simulink model "Research_project_CSTR_cascade"  (R2022b)
settings: Solver=ode23s  StartTime=0.0  StopTime=360  RelTol=1e-3
model workspace (MAT data in the model file):
  Var = 0
undefined symbols (not defined in the file): A, CA0, FA0, Tfeed, Tfeedout, Tj, U, V, v0, Xin, Xout
(part 1 of 2)
settings Model: Creator=ep740  LastModifiedBy=ep740

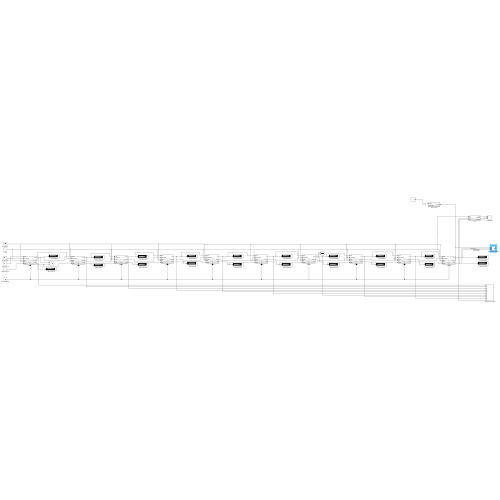
[thumbnail: Simulink's stored preview of the top-level diagram]
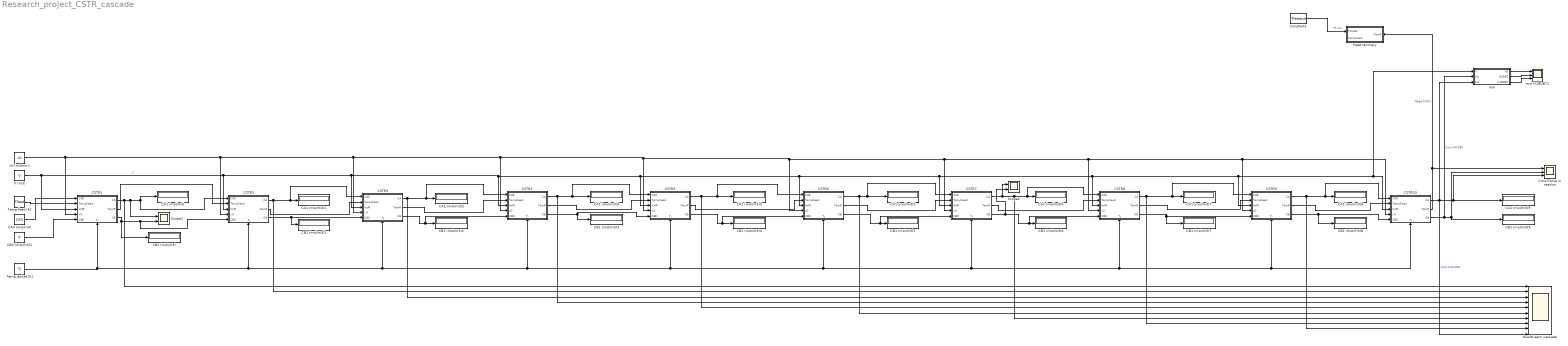
== system Research_project_CSTR_cascade ==
  CA0 (mol/m3) : Constant  Value=CA0
  CA1 (mol/m3){,1..9} (10 alike) : Display
  CB0 (mol/m3)1 : Constant  Value=0
  CB1 (mol/m3){,1..9} (10 alike) : Display
  CSTR1 : Subsystem
      settings: PortSchema="{\"entries\":[{\"content\":{\"sides\":[{\"content\":{\"connectorIds\":[\"In1\",\"In2\",\"In3\",\"In4\",\"In5\"]},\"type\":\"ConnectorPlacement.EquallySpacedRectSide\",\"uuid\":\"eea4af67-33e6-4bfc-a396-c7a4a079851b\"},{\"content\":{\"connectorIds\":[\"Out1\",\"Out2\",\"Out3\"],\"side\":\"RIGHT\"},\"type\":\"ConnectorPlacement.EquallySpacedRectSide\",\"uuid\":\"f422c120-f512-47db-9acf-190dfdbb71b1\"},{\"content\":{\"connectorIds\":[],\"side\":\"TOP\"},\"type\":\"ConnectorPlacement.EquallySpacedRectSide\",\"uuid\":\"a25ad9e8-8239-4679-905d-cedaf00f41ce\"},{\"content\":{\"connectorIds\":[\"In6\"],\"side\":\"BOTTOM\"},\"type\":\"ConnectorPlacement.EquallySpacedRectSide\",\"uuid\":\"a59362ac-e6e7-47b6-87e1-dd90c06e84db\"}]},\"type\":\"ConnectorPlacement.EquallySpacedConnector\",\"uuid\":\"827fa9d5-9d21-4e75-ac02-d0df13947b6d\"}],\"packageUris\":[\"http://schema.mathworks.com/mf0/Connector/R2020b\"],\"version\":\"1.0\"}"
  CSTR10 : Subsystem
      settings: PortSchema="{\"entries\":[{\"content\":{\"sides\":[{\"content\":{\"connectorIds\":[\"In1\",\"In2\",\"In3\",\"In4\",\"In5\"]},\"type\":\"ConnectorPlacement.EquallySpacedRectSide\",\"uuid\":\"eea4af67-33e6-4bfc-a396-c7a4a079851b\"},{\"content\":{\"connectorIds\":[\"Out1\",\"Out2\",\"Out3\"],\"side\":\"RIGHT\"},\"type\":\"ConnectorPlacement.EquallySpacedRectSide\",\"uuid\":\"f422c120-f512-47db-9acf-190dfdbb71b1\"},{\"content\":{\"connectorIds\":[],\"side\":\"TOP\"},\"type\":\"ConnectorPlacement.EquallySpacedRectSide\",\"uuid\":\"a25ad9e8-8239-4679-905d-cedaf00f41ce\"},{\"content\":{\"connectorIds\":[\"In6\"],\"side\":\"BOTTOM\"},\"type\":\"ConnectorPlacement.EquallySpacedRectSide\",\"uuid\":\"a59362ac-e6e7-47b6-87e1-dd90c06e84db\"}]},\"type\":\"ConnectorPlacement.EquallySpacedConnector\",\"uuid\":\"827fa9d5-9d21-4e75-ac02-d0df13947b6d\"}],\"packageUris\":[\"http://schema.mathworks.com/mf0/Connector/R2020b\"],\"version\":\"1.0\"}"
  CSTR2 : Subsystem
      settings: PortSchema="{\"entries\":[{\"content\":{\"sides\":[{\"content\":{\"connectorIds\":[\"In1\",\"In2\",\"In3\",\"In4\",\"In5\"]},\"type\":\"ConnectorPlacement.EquallySpacedRectSide\",\"uuid\":\"eea4af67-33e6-4bfc-a396-c7a4a079851b\"},{\"content\":{\"connectorIds\":[\"Out1\",\"Out2\",\"Out3\"],\"side\":\"RIGHT\"},\"type\":\"ConnectorPlacement.EquallySpacedRectSide\",\"uuid\":\"f422c120-f512-47db-9acf-190dfdbb71b1\"},{\"content\":{\"connectorIds\":[],\"side\":\"TOP\"},\"type\":\"ConnectorPlacement.EquallySpacedRectSide\",\"uuid\":\"a25ad9e8-8239-4679-905d-cedaf00f41ce\"},{\"content\":{\"connectorIds\":[\"In6\"],\"side\":\"BOTTOM\"},\"type\":\"ConnectorPlacement.EquallySpacedRectSide\",\"uuid\":\"a59362ac-e6e7-47b6-87e1-dd90c06e84db\"}]},\"type\":\"ConnectorPlacement.EquallySpacedConnector\",\"uuid\":\"827fa9d5-9d21-4e75-ac02-d0df13947b6d\"}],\"packageUris\":[\"http://schema.mathworks.com/mf0/Connector/R2020b\"],\"version\":\"1.0\"}"
  CSTR3 : Subsystem
      settings: PortSchema="{\"entries\":[{\"content\":{\"sides\":[{\"content\":{\"connectorIds\":[\"In1\",\"In2\",\"In3\",\"In4\",\"In5\"]},\"type\":\"ConnectorPlacement.EquallySpacedRectSide\",\"uuid\":\"eea4af67-33e6-4bfc-a396-c7a4a079851b\"},{\"content\":{\"connectorIds\":[\"Out1\",\"Out2\",\"Out3\"],\"side\":\"RIGHT\"},\"type\":\"ConnectorPlacement.EquallySpacedRectSide\",\"uuid\":\"f422c120-f512-47db-9acf-190dfdbb71b1\"},{\"content\":{\"connectorIds\":[],\"side\":\"TOP\"},\"type\":\"ConnectorPlacement.EquallySpacedRectSide\",\"uuid\":\"a25ad9e8-8239-4679-905d-cedaf00f41ce\"},{\"content\":{\"connectorIds\":[\"In6\"],\"side\":\"BOTTOM\"},\"type\":\"ConnectorPlacement.EquallySpacedRectSide\",\"uuid\":\"a59362ac-e6e7-47b6-87e1-dd90c06e84db\"}]},\"type\":\"ConnectorPlacement.EquallySpacedConnector\",\"uuid\":\"827fa9d5-9d21-4e75-ac02-d0df13947b6d\"}],\"packageUris\":[\"http://schema.mathworks.com/mf0/Connector/R2020b\"],\"version\":\"1.0\"}"
  CSTR4 : Subsystem
      settings: PortSchema="{\"entries\":[{\"content\":{\"sides\":[{\"content\":{\"connectorIds\":[\"In1\",\"In2\",\"In3\",\"In4\",\"In5\"]},\"type\":\"ConnectorPlacement.EquallySpacedRectSide\",\"uuid\":\"eea4af67-33e6-4bfc-a396-c7a4a079851b\"},{\"content\":{\"connectorIds\":[\"Out1\",\"Out2\",\"Out3\"],\"side\":\"RIGHT\"},\"type\":\"ConnectorPlacement.EquallySpacedRectSide\",\"uuid\":\"f422c120-f512-47db-9acf-190dfdbb71b1\"},{\"content\":{\"connectorIds\":[],\"side\":\"TOP\"},\"type\":\"ConnectorPlacement.EquallySpacedRectSide\",\"uuid\":\"a25ad9e8-8239-4679-905d-cedaf00f41ce\"},{\"content\":{\"connectorIds\":[\"In6\"],\"side\":\"BOTTOM\"},\"type\":\"ConnectorPlacement.EquallySpacedRectSide\",\"uuid\":\"a59362ac-e6e7-47b6-87e1-dd90c06e84db\"}]},\"type\":\"ConnectorPlacement.EquallySpacedConnector\",\"uuid\":\"827fa9d5-9d21-4e75-ac02-d0df13947b6d\"}],\"packageUris\":[\"http://schema.mathworks.com/mf0/Connector/R2020b\"],\"version\":\"1.0\"}"
  CSTR5 : Subsystem
      settings: PortSchema="{\"entries\":[{\"content\":{\"sides\":[{\"content\":{\"connectorIds\":[\"In1\",\"In2\",\"In3\",\"In4\",\"In5\"]},\"type\":\"ConnectorPlacement.EquallySpacedRectSide\",\"uuid\":\"eea4af67-33e6-4bfc-a396-c7a4a079851b\"},{\"content\":{\"connectorIds\":[\"Out1\",\"Out2\",\"Out3\"],\"side\":\"RIGHT\"},\"type\":\"ConnectorPlacement.EquallySpacedRectSide\",\"uuid\":\"f422c120-f512-47db-9acf-190dfdbb71b1\"},{\"content\":{\"connectorIds\":[],\"side\":\"TOP\"},\"type\":\"ConnectorPlacement.EquallySpacedRectSide\",\"uuid\":\"a25ad9e8-8239-4679-905d-cedaf00f41ce\"},{\"content\":{\"connectorIds\":[\"In6\"],\"side\":\"BOTTOM\"},\"type\":\"ConnectorPlacement.EquallySpacedRectSide\",\"uuid\":\"a59362ac-e6e7-47b6-87e1-dd90c06e84db\"}]},\"type\":\"ConnectorPlacement.EquallySpacedConnector\",\"uuid\":\"827fa9d5-9d21-4e75-ac02-d0df13947b6d\"}],\"packageUris\":[\"http://schema.mathworks.com/mf0/Connector/R2020b\"],\"version\":\"1.0\"}"
  CSTR6 : Subsystem
      settings: PortSchema="{\"entries\":[{\"content\":{\"sides\":[{\"content\":{\"connectorIds\":[\"In1\",\"In2\",\"In3\",\"In4\",\"In5\"]},\"type\":\"ConnectorPlacement.EquallySpacedRectSide\",\"uuid\":\"eea4af67-33e6-4bfc-a396-c7a4a079851b\"},{\"content\":{\"connectorIds\":[\"Out1\",\"Out2\",\"Out3\"],\"side\":\"RIGHT\"},\"type\":\"ConnectorPlacement.EquallySpacedRectSide\",\"uuid\":\"f422c120-f512-47db-9acf-190dfdbb71b1\"},{\"content\":{\"connectorIds\":[],\"side\":\"TOP\"},\"type\":\"ConnectorPlacement.EquallySpacedRectSide\",\"uuid\":\"a25ad9e8-8239-4679-905d-cedaf00f41ce\"},{\"content\":{\"connectorIds\":[\"In6\"],\"side\":\"BOTTOM\"},\"type\":\"ConnectorPlacement.EquallySpacedRectSide\",\"uuid\":\"a59362ac-e6e7-47b6-87e1-dd90c06e84db\"}]},\"type\":\"ConnectorPlacement.EquallySpacedConnector\",\"uuid\":\"827fa9d5-9d21-4e75-ac02-d0df13947b6d\"}],\"packageUris\":[\"http://schema.mathworks.com/mf0/Connector/R2020b\"],\"version\":\"1.0\"}"
  CSTR7 : Subsystem
      settings: PortSchema="{\"entries\":[{\"content\":{\"sides\":[{\"content\":{\"connectorIds\":[\"In1\",\"In2\",\"In3\",\"In4\",\"In5\"]},\"type\":\"ConnectorPlacement.EquallySpacedRectSide\",\"uuid\":\"eea4af67-33e6-4bfc-a396-c7a4a079851b\"},{\"content\":{\"connectorIds\":[\"Out1\",\"Out2\",\"Out3\"],\"side\":\"RIGHT\"},\"type\":\"ConnectorPlacement.EquallySpacedRectSide\",\"uuid\":\"f422c120-f512-47db-9acf-190dfdbb71b1\"},{\"content\":{\"connectorIds\":[],\"side\":\"TOP\"},\"type\":\"ConnectorPlacement.EquallySpacedRectSide\",\"uuid\":\"a25ad9e8-8239-4679-905d-cedaf00f41ce\"},{\"content\":{\"connectorIds\":[\"In6\"],\"side\":\"BOTTOM\"},\"type\":\"ConnectorPlacement.EquallySpacedRectSide\",\"uuid\":\"a59362ac-e6e7-47b6-87e1-dd90c06e84db\"}]},\"type\":\"ConnectorPlacement.EquallySpacedConnector\",\"uuid\":\"827fa9d5-9d21-4e75-ac02-d0df13947b6d\"}],\"packageUris\":[\"http://schema.mathworks.com/mf0/Connector/R2020b\"],\"version\":\"1.0\"}"
  CSTR8 : Subsystem
      settings: PortSchema="{\"entries\":[{\"content\":{\"sides\":[{\"content\":{\"connectorIds\":[\"In1\",\"In2\",\"In3\",\"In4\",\"In5\"]},\"type\":\"ConnectorPlacement.EquallySpacedRectSide\",\"uuid\":\"eea4af67-33e6-4bfc-a396-c7a4a079851b\"},{\"content\":{\"connectorIds\":[\"Out1\",\"Out2\",\"Out3\"],\"side\":\"RIGHT\"},\"type\":\"ConnectorPlacement.EquallySpacedRectSide\",\"uuid\":\"f422c120-f512-47db-9acf-190dfdbb71b1\"},{\"content\":{\"connectorIds\":[],\"side\":\"TOP\"},\"type\":\"ConnectorPlacement.EquallySpacedRectSide\",\"uuid\":\"a25ad9e8-8239-4679-905d-cedaf00f41ce\"},{\"content\":{\"connectorIds\":[\"In6\"],\"side\":\"BOTTOM\"},\"type\":\"ConnectorPlacement.EquallySpacedRectSide\",\"uuid\":\"a59362ac-e6e7-47b6-87e1-dd90c06e84db\"}]},\"type\":\"ConnectorPlacement.EquallySpacedConnector\",\"uuid\":\"827fa9d5-9d21-4e75-ac02-d0df13947b6d\"}],\"packageUris\":[\"http://schema.mathworks.com/mf0/Connector/R2020b\"],\"version\":\"1.0\"}"
  CSTR9 : Subsystem
      settings: PortSchema="{\"entries\":[{\"content\":{\"sides\":[{\"content\":{\"connectorIds\":[\"In1\",\"In2\",\"In3\",\"In4\",\"In5\"]},\"type\":\"ConnectorPlacement.EquallySpacedRectSide\",\"uuid\":\"eea4af67-33e6-4bfc-a396-c7a4a079851b\"},{\"content\":{\"connectorIds\":[\"Out1\",\"Out2\",\"Out3\"],\"side\":\"RIGHT\"},\"type\":\"ConnectorPlacement.EquallySpacedRectSide\",\"uuid\":\"f422c120-f512-47db-9acf-190dfdbb71b1\"},{\"content\":{\"connectorIds\":[],\"side\":\"TOP\"},\"type\":\"ConnectorPlacement.EquallySpacedRectSide\",\"uuid\":\"a25ad9e8-8239-4679-905d-cedaf00f41ce\"},{\"content\":{\"connectorIds\":[\"In6\"],\"side\":\"BOTTOM\"},\"type\":\"ConnectorPlacement.EquallySpacedRectSide\",\"uuid\":\"a59362ac-e6e7-47b6-87e1-dd90c06e84db\"}]},\"type\":\"ConnectorPlacement.EquallySpacedConnector\",\"uuid\":\"827fa9d5-9d21-4e75-ac02-d0df13947b6d\"}],\"packageUris\":[\"http://schema.mathworks.com/mf0/Connector/R2020b\"],\"version\":\"1.0\"}"
  Conc/Temp in reactor : Scope  NumInputPorts=3
  Constant1 : Constant  Value=Tfeedout
  Heat recovery : Subsystem
      settings: PortSchema="{\"entries\":[{\"content\":{\"sides\":[{\"content\":{\"connectorIds\":[\"In1\",\"Out1\"]},\"type\":\"ConnectorPlacement.EquallySpacedRectSide\",\"uuid\":\"573787ca-756b-47b8-a520-c4bb68d941bf\"},{\"content\":{\"connectorIds\":[\"In2\"],\"side\":\"RIGHT\"},\"type\":\"ConnectorPlacement.EquallySpacedRectSide\",\"uuid\":\"b1db1cb3-615d-4df7-8934-c0c48918d084\"},{\"content\":{\"connectorIds\":[],\"side\":\"TOP\"},\"type\":\"ConnectorPlacement.EquallySpacedRectSide\",\"uuid\":\"ffba5464-70c2-446d-94e9-0aafb3934113\"},{\"content\":{\"connectorIds\":[],\"side\":\"BOTTOM\"},\"type\":\"ConnectorPlacement.EquallySpacedRectSide\",\"uuid\":\"d4927b64-3679-4f6a-88f6-0667a528553b\"}]},\"type\":\"ConnectorPlacement.EquallySpacedConnector\",\"uuid\":\"96bf0ad9-972e-429c-80b4-1b1cb34767e8\"}],\"packageUris\":[\"http://schema.mathworks.com/mf0/Connector/R2020b\"],\"version\":\"1.0\"}"
  Scope1 : Scope  NumInputPorts=2
  Scope2 : Scope  NumInputPorts=2
  Temp Jacket (K) : Constant  Value=Tj
  Temp feed (K) : Constant  Value=Tfeed
  V (m3) : Constant  Value=V
  dCa/dt each cascade : Scope  NumInputPorts=10
  mol : Subsystem
  mol H18DBT1 : Scope  NumInputPorts=3
  v0 (m3/min) : Constant  Value=v0  VectorParams1D=off
  wires:
  CA0 (mol/m3)/1 -> CSTR1/1(CA0)
  CB0 (mol/m3)1/1 -> CSTR1/5(CB0)
  CSTR1/1(CA) -> dCa/dt each cascade/1, CSTR2/1(CA0), CA1 (mol/m3)/1, Scope1/1
  CSTR1/3(CB) -> CB1 (mol/m3)/1, CSTR2/5(CB0), Scope1/2
  V (m3)/1 -> CSTR2/3(VolR), CSTR3/3(VolR), CSTR4/3(VolR), CSTR5/3(VolR), CSTR6/3(VolR), CSTR7/3(VolR), CSTR8/3(VolR), CSTR9/3(VolR), CSTR10/3(VolR), mol/1(V), CSTR1/3(VolR)  "V"
  v0 (m3/min)/1 -> CSTR1/4(v0), CSTR2/4(v0), CSTR3/4(v0), CSTR4/4(v0), CSTR5/4(v0), CSTR6/4(v0), CSTR7/4(v0), CSTR8/4(v0), CSTR10/4(v0), CSTR9/4(v0)
  CSTR2/1(CA) -> dCa/dt each cascade/2, CSTR3/1(CA0), CA1 (mol/m3)1/1
  CSTR2/3(CB) -> CSTR3/5(CB0), CB1 (mol/m3)1/1
  CSTR1/2(TemR) -> CSTR2/2(TempFeed)
  CSTR3/3(CB) -> CSTR4/5(CB0), CB1 (mol/m3)2/1
  CSTR3/1(CA) -> dCa/dt each cascade/3, CSTR4/1(CA0), CA1 (mol/m3)2/1
  CSTR2/2(TemR) -> CSTR3/2(TempFeed)
  CSTR3/2(TemR) -> CSTR4/2(TempFeed)
  CSTR4/1(CA) -> dCa/dt each cascade/4, CSTR5/1(CA0), CA1 (mol/m3)3/1
  CSTR4/3(CB) -> CSTR5/5(CB0), CB1 (mol/m3)3/1
  CSTR5/3(CB) -> CSTR6/5(CB0), CB1 (mol/m3)4/1
  CSTR5/1(CA) -> dCa/dt each cascade/5, CSTR6/1(CA0), CA1 (mol/m3)4/1
  CSTR4/2(TemR) -> CSTR5/2(TempFeed)
  CSTR6/3(CB) -> CSTR7/5(CB0), CB1 (mol/m3)5/1
  CSTR6/1(CA) -> dCa/dt each cascade/6, CSTR7/1(CA0), CA1 (mol/m3)5/1
  CSTR5/2(TemR) -> CSTR6/2(TempFeed)
  CSTR6/2(TemR) -> CSTR7/2(TempFeed)
  CSTR7/1(CA) -> Scope2/1, dCa/dt each cascade/7, CSTR8/1(CA0), CA1 (mol/m3)6/1
  CSTR7/3(CB) -> Scope2/2, CSTR8/5(CB0), CB1 (mol/m3)6/1
  CSTR8/1(CA) -> dCa/dt each cascade/8, CSTR9/1(CA0), CA1 (mol/m3)7/1
  CSTR8/3(CB) -> CSTR9/5(CB0), CB1 (mol/m3)7/1
  CSTR7/2(TemR) -> CSTR8/2(TempFeed)
  CSTR9/3(CB) -> CSTR10/5(CB0), CB1 (mol/m3)8/1
  CSTR9/1(CA) -> dCa/dt each cascade/9, CSTR10/1(CA0), CA1 (mol/m3)8/1
  CSTR8/2(TemR) -> CSTR9/2(TempFeed)
  CSTR10/3(CB) -> mol/2(Cb), Conc/Temp in reactor/2, CB1 (mol/m3)9/1  "Conc H0-DBT"
  CSTR10/1(CA) -> mol/3(CA), dCa/dt each cascade/10, Conc/Temp in reactor/3, CA1 (mol/m3)9/1  "Conc H18-DBT"
  CSTR9/2(TemR) -> CSTR10/2(TempFeed)
  Temp Jacket (K)/1 -> CSTR2/6(Tj), CSTR3/6(Tj), CSTR4/6(Tj), CSTR5/6(Tj), CSTR6/6(Tj), CSTR7/6(Tj), CSTR8/6(Tj), CSTR10/6(Tj), CSTR9/6(Tj), CSTR1/6(Tj)
  CSTR10/2(TemR) -> Heat recovery/2(TemR), Conc/Temp in reactor/1  "Tfeed 573K)"
  Constant1/1 -> Heat recovery/1(Toutlet)  "Tf out"
  Temp feed (K)/1 -> CSTR1/2(TempFeed)
  mol/1(H2) -> mol H18DBT1/1
  mol/2(H0DBT) -> mol H18DBT1/2
  mol/3(H18DBT) -> mol H18DBT1/3

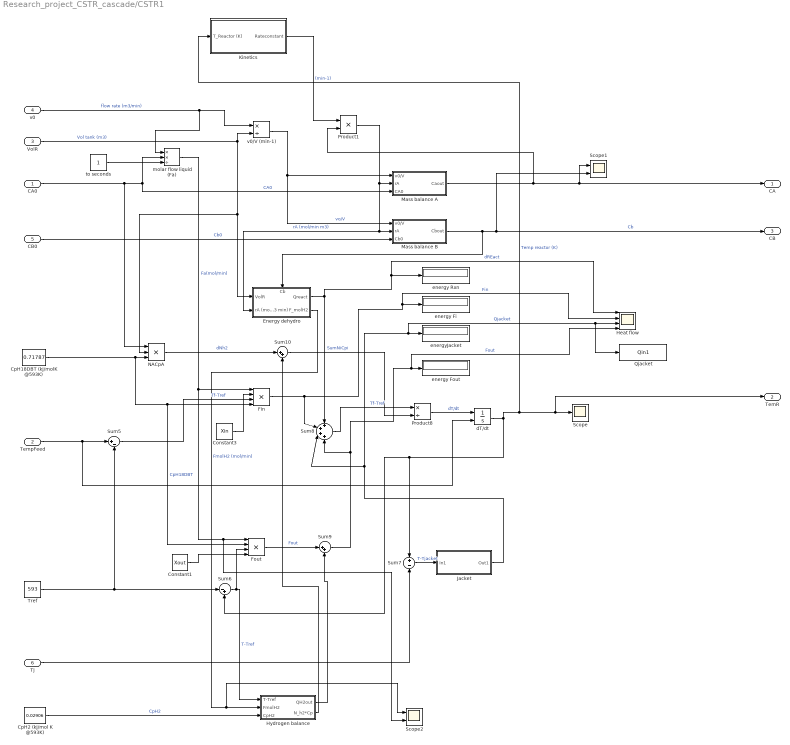
== system Research_project_CSTR_cascade/CSTR1 ==
  CA0 : Inport
  TempFeed : Inport  Port=2
  VolR : Inport  Port=3
  v0 : Inport  Port=4
  CB0 : Inport  Port=5
  Tj : Inport  Port=6
  Constant1 : Constant  Value=Xout
  Constant3 : Constant  Value=Xin
  CpH18DBT (kj/molK @593K) : Constant  Value=0.71787
  CpH2 (kj/mol K @593K) : Constant  Value=0.02906
  Energy dehydro : Subsystem
      settings: PortSchema="{\"entries\":[{\"content\":{\"sides\":[{\"content\":{\"connectorIds\":[\"In1\",\"In2\"]},\"type\":\"ConnectorPlacement.EquallySpacedRectSide\",\"uuid\":\"ea2ca829-97b9-403b-8ba1-0454ae3e30fe\"},{\"content\":{\"connectorIds\":[\"Out1\",\"Out2\"],\"side\":\"RIGHT\"},\"type\":\"ConnectorPlacement.EquallySpacedRectSide\",\"uuid\":\"58c9b242-3f0e-4d7f-8153-41ceacc042f7\"},{\"content\":{\"connectorIds\":[\"In3\"],\"side\":\"TOP\"},\"type\":\"ConnectorPlacement.EquallySpacedRectSide\",\"uuid\":\"130a98c9-d360-4861-8a60-9ab6de0c7020\"}]},\"type\":\"ConnectorPlacement.EquallySpacedConnector\",\"uuid\":\"a36fbf0c-f6b7-4cf9-83b8-7faebe270894\"}],\"packageUris\":[\"http://schema.mathworks.com/mf0/Connector/R2020b\"],\"version\":\"1.0\"}"
  Fin : Product  Inputs=4
  Fout : Product  Inputs=4
  Heat flow : Scope  NumInputPorts=4
  Hydrogen balance : Subsystem
  Jacket : Subsystem
  Kinetics : Subsystem
  Mass balance A : Subsystem
  Mass balance B : Subsystem
  NACpA : Product  Inputs=3
  Product1 : Product
  Product8 : Product  Inputs=*/
  Qjacket : ToWorkspace  VariableName=Qin1  SaveFormat=Timeseries  SampleTime=1
  Scope : Scope
  Scope1 : Scope  NumInputPorts=2
  Scope2 : Scope  NumInputPorts=2
  Sum10 : Sum  Inputs=|++
  Sum5 : Sum  Inputs=|+-
  Sum6 : Sum  Inputs=|-+
  Sum7 : Sum  Inputs=+-
  Sum8 : Sum  Inputs=++++
  Sum9 : Sum  Inputs=|++
  Tref : Constant  Value=593
  dT/dt : Integrator  InitialConditionSource=external  InitialCondition=593
  energy Fi : Display
  energy Fout : Display
  energy Rxn : Display
  energyJacket : Display
  molar flow liquid (Fa) : Product  Inputs=**/
  to seconds : Constant
  v0/V (min-1) : Product  Inputs=*/
  CA : Outport
  TemR : Outport  Port=2
  CB : Outport  Port=3
  wires:
  VolR/1 -> Energy dehydro/1(VolR), NACpA/2, v0/V (min-1)/2  "Vol tank (m3)"
  v0/1 -> v0/V (min-1)/1, molar flow liquid (Fa)/1  "flow rate (m3/min)"
  CA0/1 -> NACpA/1, molar flow liquid (Fa)/2, Mass balance A/3(CA0)  "CA0"
  Product1/1 -> Mass balance A/2(rA), Energy dehydro/2(rA (mol/m3 min)), Mass balance B/2(rA)  "rA (mol/min m3)"
  CB0/1 -> Mass balance B/3(Cb0)  "Cb0"
  v0/V (min-1)/1 -> Mass balance B/1(v0/V), Mass balance A/1(v0/V)  "vo/V"
  Mass balance B/1(Cbout) -> CB/1, Scope1/2, Energy dehydro/3(Cb)  "Cb"
  CpH18DBT (kj/molK @593K)/1 -> NACpA/3, Fin/4, Fout/2  "CpH18DBT"
  Tref/1 -> Sum5/2, Sum6/1
  Sum5/1 -> Fin/3  "Tf-Tref"
  to seconds/1 -> molar flow liquid (Fa)/3
  molar flow liquid (Fa)/1 -> Scope2/2, Fout/1, Fin/1  "Fa(mol/min)"
  dT/dt/1 -> Kinetics/1(T_Reactor (K)), TemR/1, Scope/1, Sum6/2, Sum7/1  "Temp reactor (K)"
  Sum6/1 -> Hydrogen balance/1(T-Tref), Fout/3  "T-Tref"
  Tj/1 -> Sum7/2
  Jacket/1(Out1) -> Qjacket/1, Heat flow/3, energyJacket/1, Sum8/3  "Qjacket"
  Fin/1 -> Heat flow/2, energy Fi/1, Sum8/2  "Fin"
  Sum9/1 -> Heat flow/4, energy Fout/1, Sum8/4  "Fout"
  Energy dehydro/1(Qreact) -> Sum8/1, Heat flow/1, energy Rxn/1  "dREact"
  Sum8/1 -> Product8/1  "Tf-Tref"
  Product8/1 -> dT/dt/1  "dT/dt"
  Constant1/1 -> Fout/4
  TempFeed/1 -> dT/dt/2, Sum5/1
  Kinetics/1(Rateconstant) -> Product1/1  "(min-1)"
  Constant3/1 -> Fin/2
  CpH2 (kj/mol K @593K)/1 -> Hydrogen balance/3(CpH2)  "CpH2"
  Energy dehydro/2(F_molH2) -> Scope2/1, Hydrogen balance/2(FmolH2)  "FmolH2 (mol/min)"
  Fout/1 -> Sum9/1  "Fout"
  Sum7/1 -> Jacket/1(In1)  "T-Tjacket"
  Hydrogen balance/1(QH2out) -> Sum9/2
  NACpA/1 -> Sum10/1  "dNh2"
  Sum10/1 -> Product8/2  "SumNiCpi"
  Hydrogen balance/2(N_h2*Cp) -> Sum10/2
  Mass balance A/1(Caout) -> Scope1/1, CA/1, Product1/2

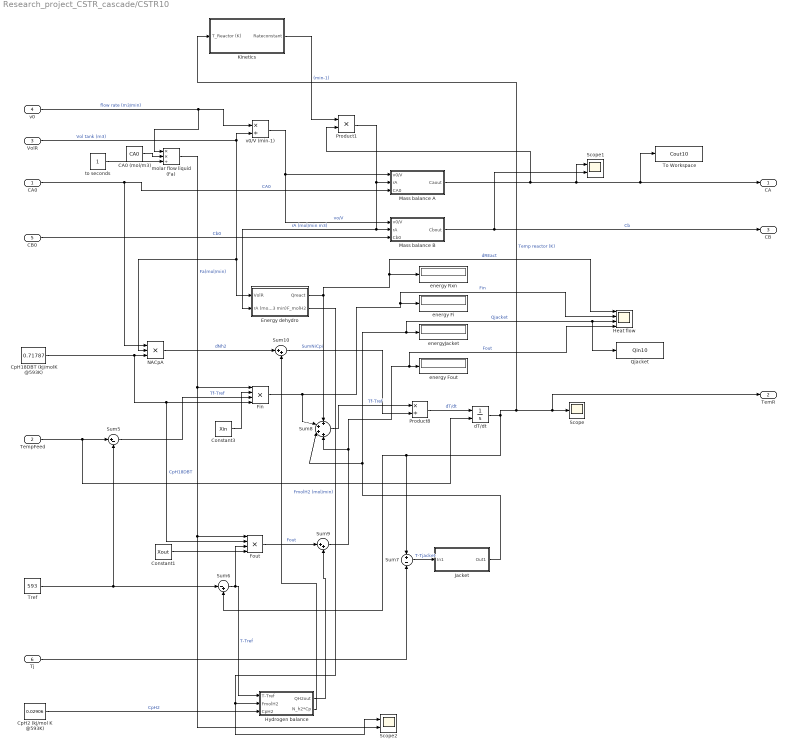
== system Research_project_CSTR_cascade/CSTR10 ==
  CA0 : Inport
  TempFeed : Inport  Port=2
  VolR : Inport  Port=3
  v0 : Inport  Port=4
  CB0 : Inport  Port=5
  Tj : Inport  Port=6
  CA0 (mol/m3) : Constant  Value=CA0
  Constant1 : Constant  Value=Xout
  Constant3 : Constant  Value=Xin
  CpH18DBT (kj/molK @593K) : Constant  Value=0.71787
  CpH2 (kj/mol K @593K) : Constant  Value=0.02906
  Energy dehydro : Subsystem
  Fin : Product  Inputs=4
  Fout : Product  Inputs=4
  Heat flow : Scope  NumInputPorts=4
  Hydrogen balance : Subsystem
  Jacket : Subsystem
  Kinetics : Subsystem
  Mass balance A : Subsystem
  Mass balance B : Subsystem
  NACpA : Product  Inputs=3
  Product1 : Product
  Product8 : Product  Inputs=*/
  Qjacket : ToWorkspace  VariableName=Qin10  SaveFormat=Timeseries  SampleTime=1
  Scope : Scope
  Scope1 : Scope  NumInputPorts=2
  Scope2 : Scope  NumInputPorts=2
  Sum10 : Sum  Inputs=|++
  Sum5 : Sum  Inputs=|+-
  Sum6 : Sum  Inputs=|-+
  Sum7 : Sum  Inputs=+-
  Sum8 : Sum  Inputs=++++
  Sum9 : Sum  Inputs=|++
  To Workspace : ToWorkspace  VariableName=Cout10  SaveFormat=Timeseries  SampleTime=5
  Tref : Constant  Value=593
  dT/dt : Integrator  InitialConditionSource=external  InitialCondition=593
  energy Fi : Display
  energy Fout : Display
  energy Rxn : Display
  energyJacket : Display
  molar flow liquid (Fa) : Product  Inputs=**/
  to seconds : Constant
  v0/V (min-1) : Product  Inputs=*/
  CA : Outport
  TemR : Outport  Port=2
  CB : Outport  Port=3
  wires:
  VolR/1 -> Energy dehydro/1(VolR), NACpA/2, v0/V (min-1)/2  "Vol tank (m3)"
  v0/1 -> v0/V (min-1)/1, molar flow liquid (Fa)/1  "flow rate (m3/min)"
  CA0/1 -> NACpA/1, Mass balance A/3(CA0)  "CA0"
  Product1/1 -> Mass balance A/2(rA), Energy dehydro/2(rA (mol/m3 min)), Mass balance B/2(rA)  "rA (mol/min m3)"
  CB0/1 -> Mass balance B/3(Cb0)  "Cb0"
  v0/V (min-1)/1 -> Mass balance B/1(v0/V), Mass balance A/1(v0/V)  "vo/V"
  Mass balance B/1(Cbout) -> CB/1, Scope1/2  "Cb"
  CpH18DBT (kj/molK @593K)/1 -> NACpA/3, Fin/4, Fout/2  "CpH18DBT"
  Tref/1 -> Sum5/2, Sum6/1
  Sum5/1 -> Fin/3  "Tf-Tref"
  to seconds/1 -> molar flow liquid (Fa)/3
  dT/dt/1 -> Kinetics/1(T_Reactor (K)), TemR/1, Scope/1, Sum6/2, Sum7/1  "Temp reactor (K)"
  Sum6/1 -> Hydrogen balance/1(T-Tref), Fout/3  "T-Tref"
  Tj/1 -> Sum7/2
  Jacket/1(Out1) -> Qjacket/1, Heat flow/3, energyJacket/1, Sum8/3  "Qjacket"
  Fin/1 -> Heat flow/2, energy Fi/1, Sum8/2  "Fin"
  Sum9/1 -> Heat flow/4, energy Fout/1, Sum8/4  "Fout"
  Energy dehydro/1(Qreact) -> Sum8/1, Heat flow/1, energy Rxn/1  "dREact"
  Sum8/1 -> Product8/1  "Tf-Tref"
  Product8/1 -> dT/dt/1  "dT/dt"
  Constant1/1 -> Fout/4
  TempFeed/1 -> dT/dt/2, Sum5/1
  Kinetics/1(Rateconstant) -> Product1/1  "(min-1)"
  Constant3/1 -> Fin/2
  CpH2 (kj/mol K @593K)/1 -> Hydrogen balance/3(CpH2)  "CpH2"
  Energy dehydro/2(F_molH2) -> Scope2/1, Hydrogen balance/2(FmolH2)  "FmolH2 (mol/min)"
  Fout/1 -> Sum9/1  "Fout"
  Sum7/1 -> Jacket/1(In1)  "T-Tjacket"
  Hydrogen balance/1(QH2out) -> Sum9/2
  NACpA/1 -> Sum10/1  "dNh2"
  Sum10/1 -> Product8/2  "SumNiCpi"
  Hydrogen balance/2(N_h2*Cp) -> Sum10/2
  Mass balance A/1(Caout) -> Scope1/1, To Workspace/1, CA/1, Product1/2
  CA0 (mol/m3)/1 -> molar flow liquid (Fa)/2
  molar flow liquid (Fa)/1 -> Fin/1, Fout/1, Scope2/2  "Fa(mol/min)"

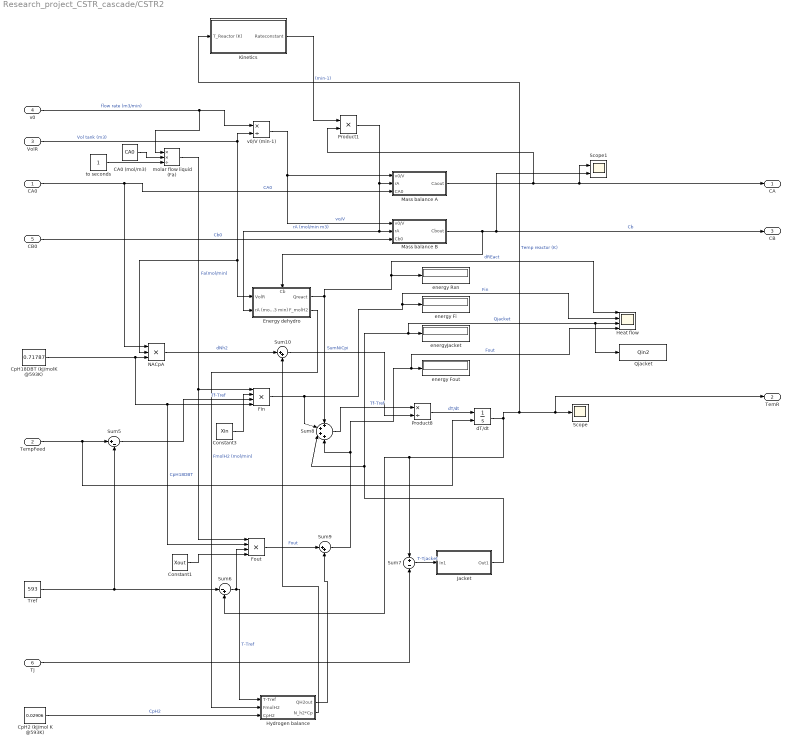
== system Research_project_CSTR_cascade/CSTR2 ==
  CA0 : Inport
  TempFeed : Inport  Port=2
  VolR : Inport  Port=3
  v0 : Inport  Port=4
  CB0 : Inport  Port=5
  Tj : Inport  Port=6
  CA0 (mol/m3) : Constant  Value=CA0
  Constant1 : Constant  Value=Xout
  Constant3 : Constant  Value=Xin
  CpH18DBT (kj/molK @593K) : Constant  Value=0.71787
  CpH2 (kj/mol K @593K) : Constant  Value=0.02906
  Energy dehydro : Subsystem
      settings: PortSchema="{\"entries\":[{\"content\":{\"sides\":[{\"content\":{\"connectorIds\":[\"In1\",\"In2\"]},\"type\":\"ConnectorPlacement.EquallySpacedRectSide\",\"uuid\":\"ea2ca829-97b9-403b-8ba1-0454ae3e30fe\"},{\"content\":{\"connectorIds\":[\"Out1\",\"Out2\"],\"side\":\"RIGHT\"},\"type\":\"ConnectorPlacement.EquallySpacedRectSide\",\"uuid\":\"58c9b242-3f0e-4d7f-8153-41ceacc042f7\"},{\"content\":{\"connectorIds\":[\"In3\"],\"side\":\"TOP\"},\"type\":\"ConnectorPlacement.EquallySpacedRectSide\",\"uuid\":\"130a98c9-d360-4861-8a60-9ab6de0c7020\"}]},\"type\":\"ConnectorPlacement.EquallySpacedConnector\",\"uuid\":\"a36fbf0c-f6b7-4cf9-83b8-7faebe270894\"}],\"packageUris\":[\"http://schema.mathworks.com/mf0/Connector/R2020b\"],\"version\":\"1.0\"}"
  Fin : Product  Inputs=4
  Fout : Product  Inputs=4
  Heat flow : Scope  NumInputPorts=4
  Hydrogen balance : Subsystem
  Jacket : Subsystem
  Kinetics : Subsystem
  Mass balance A : Subsystem
  Mass balance B : Subsystem
  NACpA : Product  Inputs=3
  Product1 : Product
  Product8 : Product  Inputs=*/
  Qjacket : ToWorkspace  VariableName=Qin2  SaveFormat=Timeseries  SampleTime=1
  Scope : Scope
  Scope1 : Scope  NumInputPorts=2
  Sum10 : Sum  Inputs=|++
  Sum5 : Sum  Inputs=|+-
  Sum6 : Sum  Inputs=|-+
  Sum7 : Sum  Inputs=+-
  Sum8 : Sum  Inputs=++++
  Sum9 : Sum  Inputs=|++
  Tref : Constant  Value=593
  dT/dt : Integrator  InitialConditionSource=external  InitialCondition=593
  energy Fi : Display
  energy Fout : Display
  energy Rxn : Display
  energyJacket : Display
  molar flow liquid (Fa) : Product  Inputs=**/
  to seconds : Constant
  v0/V (min-1) : Product  Inputs=*/
  CA : Outport
  TemR : Outport  Port=2
  CB : Outport  Port=3
  wires:
  VolR/1 -> Energy dehydro/1(VolR), NACpA/2, v0/V (min-1)/2  "Vol tank (m3)"
  v0/1 -> v0/V (min-1)/1, molar flow liquid (Fa)/1  "flow rate (m3/min)"
  CA0/1 -> NACpA/1, Mass balance A/3(CA0)  "CA0"
  Product1/1 -> Mass balance A/2(rA), Energy dehydro/2(rA (mol/m3 min)), Mass balance B/2(rA)  "rA (mol/min m3)"
  CB0/1 -> Mass balance B/3(Cb0)  "Cb0"
  v0/V (min-1)/1 -> Mass balance B/1(v0/V), Mass balance A/1(v0/V)  "vo/V"
  Mass balance B/1(Cbout) -> CB/1, Scope1/2, Energy dehydro/3(Cb)  "Cb"
  CpH18DBT (kj/molK @593K)/1 -> NACpA/3, Fin/4, Fout/2  "CpH18DBT"
  Tref/1 -> Sum5/2, Sum6/1
  Sum5/1 -> Fin/3  "Tf-Tref"
  to seconds/1 -> molar flow liquid (Fa)/3
  molar flow liquid (Fa)/1 -> Fout/1, Fin/1  "Fa(mol/min)"
  dT/dt/1 -> Kinetics/1(T_Reactor (K)), TemR/1, Scope/1, Sum6/2, Sum7/1  "Temp reactor (K)"
  Sum6/1 -> Hydrogen balance/1(T-Tref), Fout/3  "T-Tref"
  Tj/1 -> Sum7/2
  Jacket/1(Out1) -> Qjacket/1, Heat flow/3, energyJacket/1, Sum8/3  "Qjacket"
  Fin/1 -> Heat flow/2, energy Fi/1, Sum8/2  "Fin"
  Sum9/1 -> Heat flow/4, energy Fout/1, Sum8/4  "Fout"
  Energy dehydro/1(Qreact) -> Sum8/1, Heat flow/1, energy Rxn/1  "dREact"
  Sum8/1 -> Product8/1  "Tf-Tref"
  Product8/1 -> dT/dt/1  "dT/dt"
  Constant1/1 -> Fout/4
  TempFeed/1 -> dT/dt/2, Sum5/1
  Kinetics/1(Rateconstant) -> Product1/1  "(min-1)"
  Constant3/1 -> Fin/2
  CpH2 (kj/mol K @593K)/1 -> Hydrogen balance/3(CpH2)  "CpH2"
  Energy dehydro/2(F_molH2) -> Hydrogen balance/2(FmolH2)  "FmolH2 (mol/min)"
  Fout/1 -> Sum9/1  "Fout"
  Sum7/1 -> Jacket/1(In1)  "T-Tjacket"
  Hydrogen balance/1(QH2out) -> Sum9/2
  NACpA/1 -> Sum10/1  "dNh2"
  Sum10/1 -> Product8/2  "SumNiCpi"
  Hydrogen balance/2(N_h2*Cp) -> Sum10/2
  Mass balance A/1(Caout) -> Scope1/1, CA/1, Product1/2
  CA0 (mol/m3)/1 -> molar flow liquid (Fa)/2

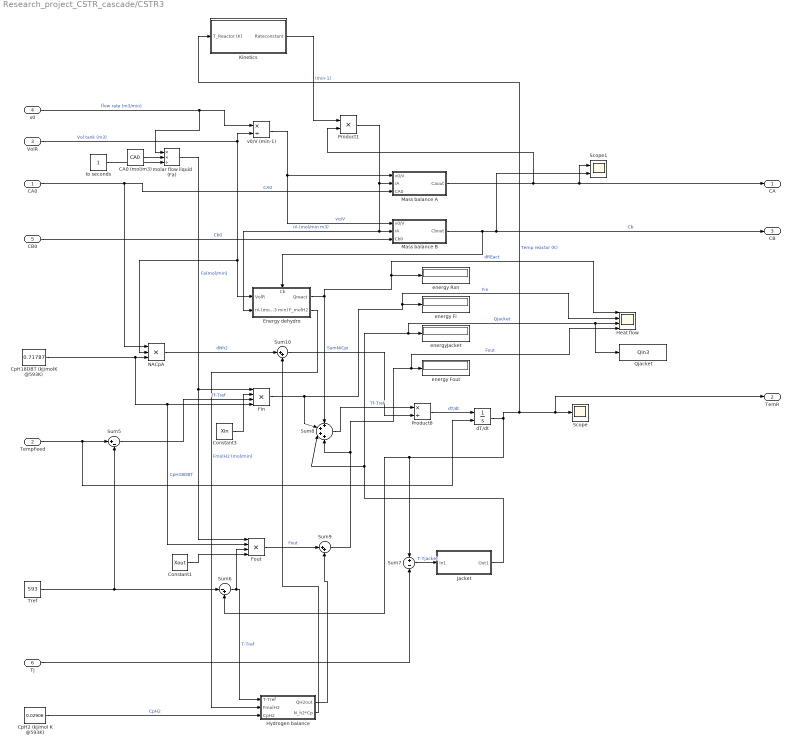
== system Research_project_CSTR_cascade/CSTR3 ==
  CA0 : Inport
  TempFeed : Inport  Port=2
  VolR : Inport  Port=3
  v0 : Inport  Port=4
  CB0 : Inport  Port=5
  Tj : Inport  Port=6
  CA0 (mol/m3) : Constant  Value=CA0
  Constant1 : Constant  Value=Xout
  Constant3 : Constant  Value=Xin
  CpH18DBT (kj/molK @593K) : Constant  Value=0.71787
  CpH2 (kj/mol K @593K) : Constant  Value=0.02906
  Energy dehydro : Subsystem
      settings: PortSchema="{\"entries\":[{\"content\":{\"sides\":[{\"content\":{\"connectorIds\":[\"In1\",\"In2\"]},\"type\":\"ConnectorPlacement.EquallySpacedRectSide\",\"uuid\":\"ea2ca829-97b9-403b-8ba1-0454ae3e30fe\"},{\"content\":{\"connectorIds\":[\"Out1\",\"Out2\"],\"side\":\"RIGHT\"},\"type\":\"ConnectorPlacement.EquallySpacedRectSide\",\"uuid\":\"58c9b242-3f0e-4d7f-8153-41ceacc042f7\"},{\"content\":{\"connectorIds\":[\"In3\"],\"side\":\"TOP\"},\"type\":\"ConnectorPlacement.EquallySpacedRectSide\",\"uuid\":\"130a98c9-d360-4861-8a60-9ab6de0c7020\"}]},\"type\":\"ConnectorPlacement.EquallySpacedConnector\",\"uuid\":\"a36fbf0c-f6b7-4cf9-83b8-7faebe270894\"}],\"packageUris\":[\"http://schema.mathworks.com/mf0/Connector/R2020b\"],\"version\":\"1.0\"}"
  Fin : Product  Inputs=4
  Fout : Product  Inputs=4
  Heat flow : Scope  NumInputPorts=4
  Hydrogen balance : Subsystem
  Jacket : Subsystem
  Kinetics : Subsystem
  Mass balance A : Subsystem
  Mass balance B : Subsystem
  NACpA : Product  Inputs=3
  Product1 : Product
  Product8 : Product  Inputs=*/
  Qjacket : ToWorkspace  VariableName=Qin3  SaveFormat=Timeseries  SampleTime=1
  Scope : Scope
  Scope1 : Scope  NumInputPorts=2
  Sum10 : Sum  Inputs=|++
  Sum5 : Sum  Inputs=|+-
  Sum6 : Sum  Inputs=|-+
  Sum7 : Sum  Inputs=+-
  Sum8 : Sum  Inputs=++++
  Sum9 : Sum  Inputs=|++
  Tref : Constant  Value=593
  dT/dt : Integrator  InitialConditionSource=external  InitialCondition=593
  energy Fi : Display
  energy Fout : Display
  energy Rxn : Display
  energyJacket : Display
  molar flow liquid (Fa) : Product  Inputs=**/
  to seconds : Constant
  v0/V (min-1) : Product  Inputs=*/
  CA : Outport
  TemR : Outport  Port=2
  CB : Outport  Port=3
  wires:
  VolR/1 -> Energy dehydro/1(VolR), NACpA/2, v0/V (min-1)/2  "Vol tank (m3)"
  v0/1 -> v0/V (min-1)/1, molar flow liquid (Fa)/1  "flow rate (m3/min)"
  CA0/1 -> NACpA/1, Mass balance A/3(CA0)  "CA0"
  Product1/1 -> Mass balance A/2(rA), Energy dehydro/2(rA (mol/m3 min)), Mass balance B/2(rA)  "rA (mol/min m3)"
  CB0/1 -> Mass balance B/3(Cb0)  "Cb0"
  v0/V (min-1)/1 -> Mass balance B/1(v0/V), Mass balance A/1(v0/V)  "vo/V"
  Mass balance B/1(Cbout) -> CB/1, Scope1/2, Energy dehydro/3(Cb)  "Cb"
  CpH18DBT (kj/molK @593K)/1 -> NACpA/3, Fin/4, Fout/2  "CpH18DBT"
  Tref/1 -> Sum5/2, Sum6/1
  Sum5/1 -> Fin/3  "Tf-Tref"
  to seconds/1 -> molar flow liquid (Fa)/3
  molar flow liquid (Fa)/1 -> Fout/1, Fin/1  "Fa(mol/min)"
  dT/dt/1 -> Kinetics/1(T_Reactor (K)), TemR/1, Scope/1, Sum6/2, Sum7/1  "Temp reactor (K)"
  Sum6/1 -> Hydrogen balance/1(T-Tref), Fout/3  "T-Tref"
  Tj/1 -> Sum7/2
  Jacket/1(Out1) -> Qjacket/1, Heat flow/3, energyJacket/1, Sum8/3  "Qjacket"
  Fin/1 -> Heat flow/2, energy Fi/1, Sum8/2  "Fin"
  Sum9/1 -> Heat flow/4, energy Fout/1, Sum8/4  "Fout"
  Energy dehydro/1(Qreact) -> Sum8/1, Heat flow/1, energy Rxn/1  "dREact"
  Sum8/1 -> Product8/1  "Tf-Tref"
  Product8/1 -> dT/dt/1  "dT/dt"
  Constant1/1 -> Fout/4
  TempFeed/1 -> dT/dt/2, Sum5/1
  Kinetics/1(Rateconstant) -> Product1/1  "(min-1)"
  Constant3/1 -> Fin/2
  CpH2 (kj/mol K @593K)/1 -> Hydrogen balance/3(CpH2)  "CpH2"
  Energy dehydro/2(F_molH2) -> Hydrogen balance/2(FmolH2)  "FmolH2 (mol/min)"
  Fout/1 -> Sum9/1  "Fout"
  Sum7/1 -> Jacket/1(In1)  "T-Tjacket"
  Hydrogen balance/1(QH2out) -> Sum9/2
  NACpA/1 -> Sum10/1  "dNh2"
  Sum10/1 -> Product8/2  "SumNiCpi"
  Hydrogen balance/2(N_h2*Cp) -> Sum10/2
  Mass balance A/1(Caout) -> Scope1/1, CA/1, Product1/2
  CA0 (mol/m3)/1 -> molar flow liquid (Fa)/2

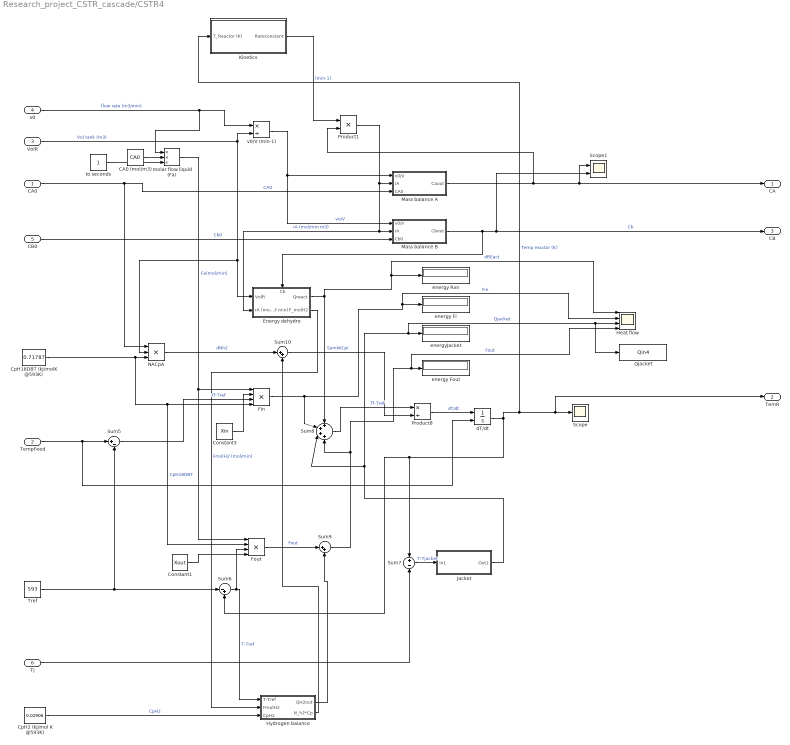
== system Research_project_CSTR_cascade/CSTR4 ==
  CA0 : Inport
  TempFeed : Inport  Port=2
  VolR : Inport  Port=3
  v0 : Inport  Port=4
  CB0 : Inport  Port=5
  Tj : Inport  Port=6
  CA0 (mol/m3) : Constant  Value=CA0
  Constant1 : Constant  Value=Xout
  Constant3 : Constant  Value=Xin
  CpH18DBT (kj/molK @593K) : Constant  Value=0.71787
  CpH2 (kj/mol K @593K) : Constant  Value=0.02906
  Energy dehydro : Subsystem
      settings: PortSchema="{\"entries\":[{\"content\":{\"sides\":[{\"content\":{\"connectorIds\":[\"In1\",\"In2\"]},\"type\":\"ConnectorPlacement.EquallySpacedRectSide\",\"uuid\":\"ea2ca829-97b9-403b-8ba1-0454ae3e30fe\"},{\"content\":{\"connectorIds\":[\"Out1\",\"Out2\"],\"side\":\"RIGHT\"},\"type\":\"ConnectorPlacement.EquallySpacedRectSide\",\"uuid\":\"58c9b242-3f0e-4d7f-8153-41ceacc042f7\"},{\"content\":{\"connectorIds\":[\"In3\"],\"side\":\"TOP\"},\"type\":\"ConnectorPlacement.EquallySpacedRectSide\",\"uuid\":\"130a98c9-d360-4861-8a60-9ab6de0c7020\"}]},\"type\":\"ConnectorPlacement.EquallySpacedConnector\",\"uuid\":\"a36fbf0c-f6b7-4cf9-83b8-7faebe270894\"}],\"packageUris\":[\"http://schema.mathworks.com/mf0/Connector/R2020b\"],\"version\":\"1.0\"}"
  Fin : Product  Inputs=4
  Fout : Product  Inputs=4
  Heat flow : Scope  NumInputPorts=4
  Hydrogen balance : Subsystem
  Jacket : Subsystem
  Kinetics : Subsystem
  Mass balance A : Subsystem
  Mass balance B : Subsystem
  NACpA : Product  Inputs=3
  Product1 : Product
  Product8 : Product  Inputs=*/
  Qjacket : ToWorkspace  VariableName=Qin4  SaveFormat=Timeseries  SampleTime=1
  Scope : Scope
  Scope1 : Scope  NumInputPorts=2
  Sum10 : Sum  Inputs=|++
  Sum5 : Sum  Inputs=|+-
  Sum6 : Sum  Inputs=|-+
  Sum7 : Sum  Inputs=+-
  Sum8 : Sum  Inputs=++++
  Sum9 : Sum  Inputs=|++
  Tref : Constant  Value=593
  dT/dt : Integrator  InitialConditionSource=external  InitialCondition=593
  energy Fi : Display
  energy Fout : Display
  energy Rxn : Display
  energyJacket : Display
  molar flow liquid (Fa) : Product  Inputs=**/
  to seconds : Constant
  v0/V (min-1) : Product  Inputs=*/
  CA : Outport
  TemR : Outport  Port=2
  CB : Outport  Port=3
  wires:
  VolR/1 -> Energy dehydro/1(VolR), NACpA/2, v0/V (min-1)/2  "Vol tank (m3)"
  v0/1 -> v0/V (min-1)/1, molar flow liquid (Fa)/1  "flow rate (m3/min)"
  CA0/1 -> NACpA/1, Mass balance A/3(CA0)  "CA0"
  Product1/1 -> Mass balance A/2(rA), Energy dehydro/2(rA (mol/m3 min)), Mass balance B/2(rA)  "rA (mol/min m3)"
  CB0/1 -> Mass balance B/3(Cb0)  "Cb0"
  v0/V (min-1)/1 -> Mass balance B/1(v0/V), Mass balance A/1(v0/V)  "vo/V"
  Mass balance B/1(Cbout) -> CB/1, Scope1/2, Energy dehydro/3(Cb)  "Cb"
  CpH18DBT (kj/molK @593K)/1 -> NACpA/3, Fin/4, Fout/2  "CpH18DBT"
  Tref/1 -> Sum5/2, Sum6/1
  Sum5/1 -> Fin/3  "Tf-Tref"
  to seconds/1 -> molar flow liquid (Fa)/3
  molar flow liquid (Fa)/1 -> Fout/1, Fin/1  "Fa(mol/min)"
  dT/dt/1 -> Kinetics/1(T_Reactor (K)), TemR/1, Scope/1, Sum6/2, Sum7/1  "Temp reactor (K)"
  Sum6/1 -> Hydrogen balance/1(T-Tref), Fout/3  "T-Tref"
  Tj/1 -> Sum7/2
  Jacket/1(Out1) -> Qjacket/1, Heat flow/3, energyJacket/1, Sum8/3  "Qjacket"
  Fin/1 -> Heat flow/2, energy Fi/1, Sum8/2  "Fin"
  Sum9/1 -> Heat flow/4, energy Fout/1, Sum8/4  "Fout"
  Energy dehydro/1(Qreact) -> Sum8/1, Heat flow/1, energy Rxn/1  "dREact"
  Sum8/1 -> Product8/1  "Tf-Tref"
  Product8/1 -> dT/dt/1  "dT/dt"
  Constant1/1 -> Fout/4
  TempFeed/1 -> dT/dt/2, Sum5/1
  Kinetics/1(Rateconstant) -> Product1/1  "(min-1)"
  Constant3/1 -> Fin/2
  CpH2 (kj/mol K @593K)/1 -> Hydrogen balance/3(CpH2)  "CpH2"
  Energy dehydro/2(F_molH2) -> Hydrogen balance/2(FmolH2)  "FmolH2 (mol/min)"
  Fout/1 -> Sum9/1  "Fout"
  Sum7/1 -> Jacket/1(In1)  "T-Tjacket"
  Hydrogen balance/1(QH2out) -> Sum9/2
  NACpA/1 -> Sum10/1  "dNh2"
  Sum10/1 -> Product8/2  "SumNiCpi"
  Hydrogen balance/2(N_h2*Cp) -> Sum10/2
  Mass balance A/1(Caout) -> Scope1/1, CA/1, Product1/2
  CA0 (mol/m3)/1 -> molar flow liquid (Fa)/2

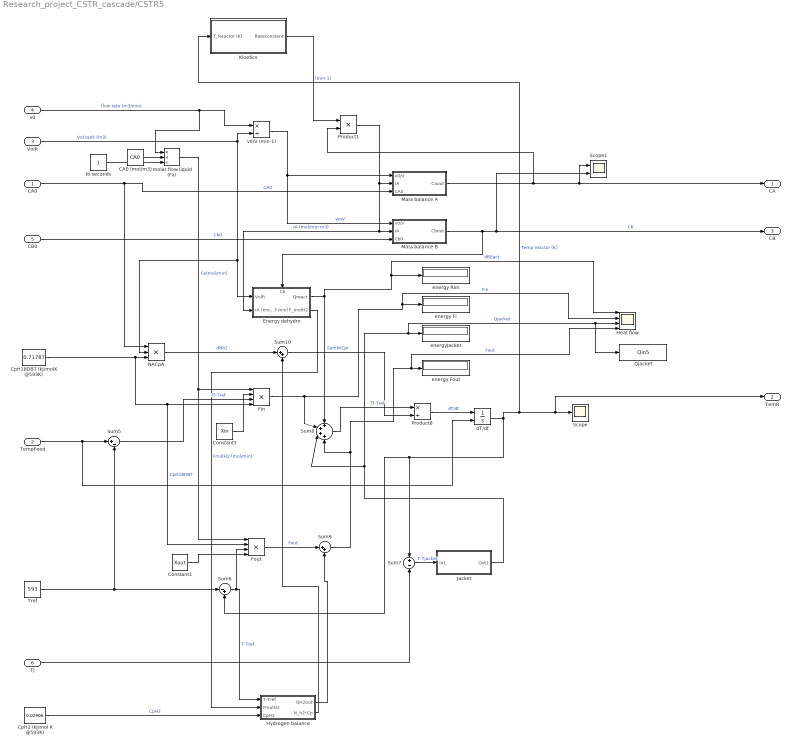
== system Research_project_CSTR_cascade/CSTR5 ==
  CA0 : Inport
  TempFeed : Inport  Port=2
  VolR : Inport  Port=3
  v0 : Inport  Port=4
  CB0 : Inport  Port=5
  Tj : Inport  Port=6
  CA0 (mol/m3) : Constant  Value=CA0
  Constant1 : Constant  Value=Xout
  Constant3 : Constant  Value=Xin
  CpH18DBT (kj/molK @593K) : Constant  Value=0.71787
  CpH2 (kj/mol K @593K) : Constant  Value=0.02906
  Energy dehydro : Subsystem
      settings: PortSchema="{\"entries\":[{\"content\":{\"sides\":[{\"content\":{\"connectorIds\":[\"In1\",\"In2\"]},\"type\":\"ConnectorPlacement.EquallySpacedRectSide\",\"uuid\":\"ea2ca829-97b9-403b-8ba1-0454ae3e30fe\"},{\"content\":{\"connectorIds\":[\"Out1\",\"Out2\"],\"side\":\"RIGHT\"},\"type\":\"ConnectorPlacement.EquallySpacedRectSide\",\"uuid\":\"58c9b242-3f0e-4d7f-8153-41ceacc042f7\"},{\"content\":{\"connectorIds\":[\"In3\"],\"side\":\"TOP\"},\"type\":\"ConnectorPlacement.EquallySpacedRectSide\",\"uuid\":\"130a98c9-d360-4861-8a60-9ab6de0c7020\"}]},\"type\":\"ConnectorPlacement.EquallySpacedConnector\",\"uuid\":\"a36fbf0c-f6b7-4cf9-83b8-7faebe270894\"}],\"packageUris\":[\"http://schema.mathworks.com/mf0/Connector/R2020b\"],\"version\":\"1.0\"}"
  Fin : Product  Inputs=4
  Fout : Product  Inputs=4
  Heat flow : Scope  NumInputPorts=4
  Hydrogen balance : Subsystem
  Jacket : Subsystem
  Kinetics : Subsystem
  Mass balance A : Subsystem
  Mass balance B : Subsystem
  NACpA : Product  Inputs=3
  Product1 : Product
  Product8 : Product  Inputs=*/
  Qjacket : ToWorkspace  VariableName=Qin5  SaveFormat=Timeseries  SampleTime=1
  Scope : Scope
  Scope1 : Scope  NumInputPorts=2
  Sum10 : Sum  Inputs=|++
  Sum5 : Sum  Inputs=|+-
  Sum6 : Sum  Inputs=|-+
  Sum7 : Sum  Inputs=+-
  Sum8 : Sum  Inputs=++++
  Sum9 : Sum  Inputs=|++
  Tref : Constant  Value=593
  dT/dt : Integrator  InitialConditionSource=external  InitialCondition=593
  energy Fi : Display
  energy Fout : Display
  energy Rxn : Display
  energyJacket : Display
  molar flow liquid (Fa) : Product  Inputs=**/
  to seconds : Constant
  v0/V (min-1) : Product  Inputs=*/
  CA : Outport
  TemR : Outport  Port=2
  CB : Outport  Port=3
  wires:
  VolR/1 -> Energy dehydro/1(VolR), NACpA/2, v0/V (min-1)/2  "Vol tank (m3)"
  v0/1 -> v0/V (min-1)/1, molar flow liquid (Fa)/1  "flow rate (m3/min)"
  CA0/1 -> NACpA/1, Mass balance A/3(CA0)  "CA0"
  Product1/1 -> Mass balance A/2(rA), Energy dehydro/2(rA (mol/m3 min)), Mass balance B/2(rA)  "rA (mol/min m3)"
  CB0/1 -> Mass balance B/3(Cb0)  "Cb0"
  v0/V (min-1)/1 -> Mass balance B/1(v0/V), Mass balance A/1(v0/V)  "vo/V"
  Mass balance B/1(Cbout) -> CB/1, Scope1/2, Energy dehydro/3(Cb)  "Cb"
  CpH18DBT (kj/molK @593K)/1 -> NACpA/3, Fin/4, Fout/2  "CpH18DBT"
  Tref/1 -> Sum5/2, Sum6/1
  Sum5/1 -> Fin/3  "Tf-Tref"
  to seconds/1 -> molar flow liquid (Fa)/3
  molar flow liquid (Fa)/1 -> Fout/1, Fin/1  "Fa(mol/min)"
  dT/dt/1 -> Kinetics/1(T_Reactor (K)), TemR/1, Scope/1, Sum6/2, Sum7/1  "Temp reactor (K)"
  Sum6/1 -> Hydrogen balance/1(T-Tref), Fout/3  "T-Tref"
  Tj/1 -> Sum7/2
  Jacket/1(Out1) -> Qjacket/1, Heat flow/3, energyJacket/1, Sum8/3  "Qjacket"
  Fin/1 -> Heat flow/2, energy Fi/1, Sum8/2  "Fin"
  Sum9/1 -> Heat flow/4, energy Fout/1, Sum8/4  "Fout"
  Energy dehydro/1(Qreact) -> Sum8/1, Heat flow/1, energy Rxn/1  "dREact"
  Sum8/1 -> Product8/1  "Tf-Tref"
  Product8/1 -> dT/dt/1  "dT/dt"
  Constant1/1 -> Fout/4
  TempFeed/1 -> dT/dt/2, Sum5/1
  Kinetics/1(Rateconstant) -> Product1/1  "(min-1)"
  Constant3/1 -> Fin/2
  CpH2 (kj/mol K @593K)/1 -> Hydrogen balance/3(CpH2)  "CpH2"
  Energy dehydro/2(F_molH2) -> Hydrogen balance/2(FmolH2)  "FmolH2 (mol/min)"
  Fout/1 -> Sum9/1  "Fout"
  Sum7/1 -> Jacket/1(In1)  "T-Tjacket"
  Hydrogen balance/1(QH2out) -> Sum9/2
  NACpA/1 -> Sum10/1  "dNh2"
  Sum10/1 -> Product8/2  "SumNiCpi"
  Hydrogen balance/2(N_h2*Cp) -> Sum10/2
  Mass balance A/1(Caout) -> Scope1/1, CA/1, Product1/2
  CA0 (mol/m3)/1 -> molar flow liquid (Fa)/2

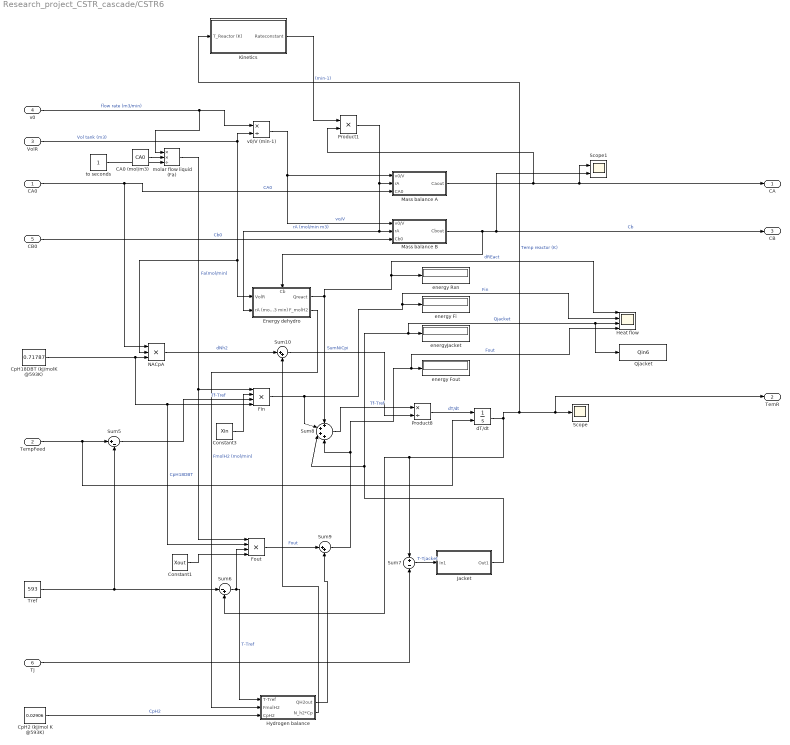
== system Research_project_CSTR_cascade/CSTR6 ==
  CA0 : Inport
  TempFeed : Inport  Port=2
  VolR : Inport  Port=3
  v0 : Inport  Port=4
  CB0 : Inport  Port=5
  Tj : Inport  Port=6
  CA0 (mol/m3) : Constant  Value=CA0
  Constant1 : Constant  Value=Xout
  Constant3 : Constant  Value=Xin
  CpH18DBT (kj/molK @593K) : Constant  Value=0.71787
  CpH2 (kj/mol K @593K) : Constant  Value=0.02906
  Energy dehydro : Subsystem
      settings: PortSchema="{\"entries\":[{\"content\":{\"sides\":[{\"content\":{\"connectorIds\":[\"In1\",\"In2\"]},\"type\":\"ConnectorPlacement.EquallySpacedRectSide\",\"uuid\":\"ea2ca829-97b9-403b-8ba1-0454ae3e30fe\"},{\"content\":{\"connectorIds\":[\"Out1\",\"Out2\"],\"side\":\"RIGHT\"},\"type\":\"ConnectorPlacement.EquallySpacedRectSide\",\"uuid\":\"58c9b242-3f0e-4d7f-8153-41ceacc042f7\"},{\"content\":{\"connectorIds\":[\"In3\"],\"side\":\"TOP\"},\"type\":\"ConnectorPlacement.EquallySpacedRectSide\",\"uuid\":\"130a98c9-d360-4861-8a60-9ab6de0c7020\"}]},\"type\":\"ConnectorPlacement.EquallySpacedConnector\",\"uuid\":\"a36fbf0c-f6b7-4cf9-83b8-7faebe270894\"}],\"packageUris\":[\"http://schema.mathworks.com/mf0/Connector/R2020b\"],\"version\":\"1.0\"}"
  Fin : Product  Inputs=4
  Fout : Product  Inputs=4
  Heat flow : Scope  NumInputPorts=4
  Hydrogen balance : Subsystem
  Jacket : Subsystem
  Kinetics : Subsystem
  Mass balance A : Subsystem
  Mass balance B : Subsystem
  NACpA : Product  Inputs=3
  Product1 : Product
  Product8 : Product  Inputs=*/
  Qjacket : ToWorkspace  VariableName=Qin6  SaveFormat=Timeseries  SampleTime=1
  Scope : Scope
  Scope1 : Scope  NumInputPorts=2
  Sum10 : Sum  Inputs=|++
  Sum5 : Sum  Inputs=|+-
  Sum6 : Sum  Inputs=|-+
  Sum7 : Sum  Inputs=+-
  Sum8 : Sum  Inputs=++++
  Sum9 : Sum  Inputs=|++
  Tref : Constant  Value=593
  dT/dt : Integrator  InitialConditionSource=external  InitialCondition=593
  energy Fi : Display
  energy Fout : Display
  energy Rxn : Display
  energyJacket : Display
  molar flow liquid (Fa) : Product  Inputs=**/
  to seconds : Constant
  v0/V (min-1) : Product  Inputs=*/
  CA : Outport
  TemR : Outport  Port=2
  CB : Outport  Port=3
  wires:
  VolR/1 -> Energy dehydro/1(VolR), NACpA/2, v0/V (min-1)/2  "Vol tank (m3)"
  v0/1 -> v0/V (min-1)/1, molar flow liquid (Fa)/1  "flow rate (m3/min)"
  CA0/1 -> NACpA/1, Mass balance A/3(CA0)  "CA0"
  Product1/1 -> Mass balance A/2(rA), Energy dehydro/2(rA (mol/m3 min)), Mass balance B/2(rA)  "rA (mol/min m3)"
  CB0/1 -> Mass balance B/3(Cb0)  "Cb0"
  v0/V (min-1)/1 -> Mass balance B/1(v0/V), Mass balance A/1(v0/V)  "vo/V"
  Mass balance B/1(Cbout) -> CB/1, Scope1/2, Energy dehydro/3(Cb)  "Cb"
  CpH18DBT (kj/molK @593K)/1 -> NACpA/3, Fin/4, Fout/2  "CpH18DBT"
  Tref/1 -> Sum5/2, Sum6/1
  Sum5/1 -> Fin/3  "Tf-Tref"
  to seconds/1 -> molar flow liquid (Fa)/3
  molar flow liquid (Fa)/1 -> Fout/1, Fin/1  "Fa(mol/min)"
  dT/dt/1 -> Kinetics/1(T_Reactor (K)), TemR/1, Scope/1, Sum6/2, Sum7/1  "Temp reactor (K)"
  Sum6/1 -> Hydrogen balance/1(T-Tref), Fout/3  "T-Tref"
  Tj/1 -> Sum7/2
  Jacket/1(Out1) -> Qjacket/1, Heat flow/3, energyJacket/1, Sum8/3  "Qjacket"
  Fin/1 -> Heat flow/2, energy Fi/1, Sum8/2  "Fin"
  Sum9/1 -> Heat flow/4, energy Fout/1, Sum8/4  "Fout"
  Energy dehydro/1(Qreact) -> Sum8/1, Heat flow/1, energy Rxn/1  "dREact"
  Sum8/1 -> Product8/1  "Tf-Tref"
  Product8/1 -> dT/dt/1  "dT/dt"
  Constant1/1 -> Fout/4
  TempFeed/1 -> dT/dt/2, Sum5/1
  Kinetics/1(Rateconstant) -> Product1/1  "(min-1)"
  Constant3/1 -> Fin/2
  CpH2 (kj/mol K @593K)/1 -> Hydrogen balance/3(CpH2)  "CpH2"
  Energy dehydro/2(F_molH2) -> Hydrogen balance/2(FmolH2)  "FmolH2 (mol/min)"
  Fout/1 -> Sum9/1  "Fout"
  Sum7/1 -> Jacket/1(In1)  "T-Tjacket"
  Hydrogen balance/1(QH2out) -> Sum9/2
  NACpA/1 -> Sum10/1  "dNh2"
  Sum10/1 -> Product8/2  "SumNiCpi"
  Hydrogen balance/2(N_h2*Cp) -> Sum10/2
  Mass balance A/1(Caout) -> Scope1/1, CA/1, Product1/2
  CA0 (mol/m3)/1 -> molar flow liquid (Fa)/2

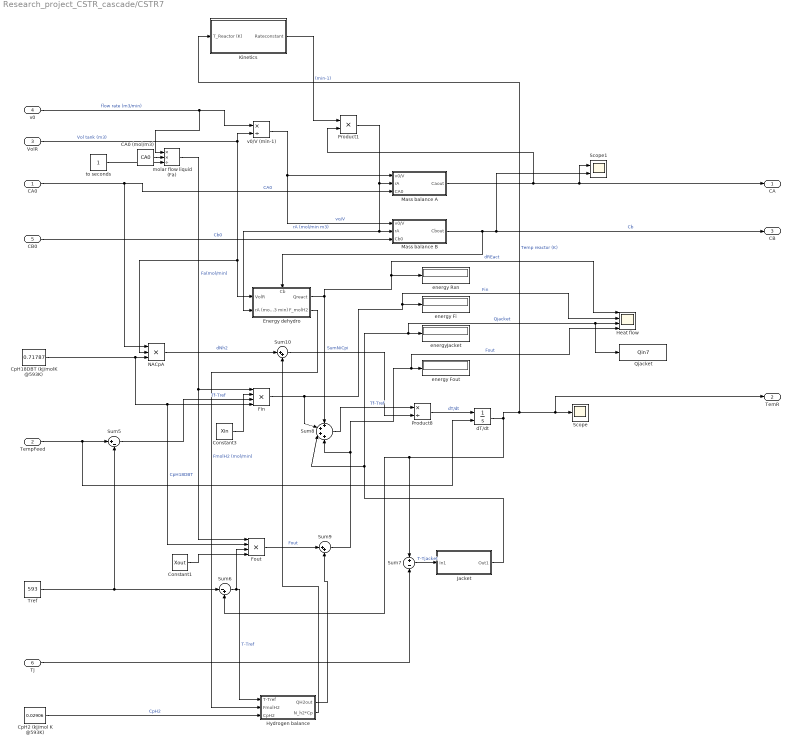
== system Research_project_CSTR_cascade/CSTR7 ==
  CA0 : Inport
  TempFeed : Inport  Port=2
  VolR : Inport  Port=3
  v0 : Inport  Port=4
  CB0 : Inport  Port=5
  Tj : Inport  Port=6
  CA0 (mol/m3) : Constant  Value=CA0
  Constant1 : Constant  Value=Xout
  Constant3 : Constant  Value=Xin
  CpH18DBT (kj/molK @593K) : Constant  Value=0.71787
  CpH2 (kj/mol K @593K) : Constant  Value=0.02906
  Energy dehydro : Subsystem
      settings: PortSchema="{\"entries\":[{\"content\":{\"sides\":[{\"content\":{\"connectorIds\":[\"In1\",\"In2\"]},\"type\":\"ConnectorPlacement.EquallySpacedRectSide\",\"uuid\":\"ea2ca829-97b9-403b-8ba1-0454ae3e30fe\"},{\"content\":{\"connectorIds\":[\"Out1\",\"Out2\"],\"side\":\"RIGHT\"},\"type\":\"ConnectorPlacement.EquallySpacedRectSide\",\"uuid\":\"58c9b242-3f0e-4d7f-8153-41ceacc042f7\"},{\"content\":{\"connectorIds\":[\"In3\"],\"side\":\"TOP\"},\"type\":\"ConnectorPlacement.EquallySpacedRectSide\",\"uuid\":\"130a98c9-d360-4861-8a60-9ab6de0c7020\"}]},\"type\":\"ConnectorPlacement.EquallySpacedConnector\",\"uuid\":\"a36fbf0c-f6b7-4cf9-83b8-7faebe270894\"}],\"packageUris\":[\"http://schema.mathworks.com/mf0/Connector/R2020b\"],\"version\":\"1.0\"}"
  Fin : Product  Inputs=4
  Fout : Product  Inputs=4
  Heat flow : Scope  NumInputPorts=4
  Hydrogen balance : Subsystem
  Jacket : Subsystem
  Kinetics : Subsystem
  Mass balance A : Subsystem
  Mass balance B : Subsystem
  NACpA : Product  Inputs=3
  Product1 : Product
  Product8 : Product  Inputs=*/
  Qjacket : ToWorkspace  VariableName=Qin7  SaveFormat=Timeseries  SampleTime=1
  Scope : Scope
  Scope1 : Scope  NumInputPorts=2
  Sum10 : Sum  Inputs=|++
  Sum5 : Sum  Inputs=|+-
  Sum6 : Sum  Inputs=|-+
  Sum7 : Sum  Inputs=+-
  Sum8 : Sum  Inputs=++++
  Sum9 : Sum  Inputs=|++
  Tref : Constant  Value=593
  dT/dt : Integrator  InitialConditionSource=external  InitialCondition=593
  energy Fi : Display
  energy Fout : Display
  energy Rxn : Display
  energyJacket : Display
  molar flow liquid (Fa) : Product  Inputs=**/
  to seconds : Constant
  v0/V (min-1) : Product  Inputs=*/
  CA : Outport
  TemR : Outport  Port=2
  CB : Outport  Port=3
  wires:
  VolR/1 -> Energy dehydro/1(VolR), NACpA/2, v0/V (min-1)/2  "Vol tank (m3)"
  v0/1 -> v0/V (min-1)/1, molar flow liquid (Fa)/1  "flow rate (m3/min)"
  CA0/1 -> NACpA/1, Mass balance A/3(CA0)  "CA0"
  Product1/1 -> Mass balance A/2(rA), Energy dehydro/2(rA (mol/m3 min)), Mass balance B/2(rA)  "rA (mol/min m3)"
  CB0/1 -> Mass balance B/3(Cb0)  "Cb0"
  v0/V (min-1)/1 -> Mass balance B/1(v0/V), Mass balance A/1(v0/V)  "vo/V"
  Mass balance B/1(Cbout) -> CB/1, Scope1/2, Energy dehydro/3(Cb)  "Cb"
  CpH18DBT (kj/molK @593K)/1 -> NACpA/3, Fin/4, Fout/2  "CpH18DBT"
  Tref/1 -> Sum5/2, Sum6/1
  Sum5/1 -> Fin/3  "Tf-Tref"
  to seconds/1 -> molar flow liquid (Fa)/3
  molar flow liquid (Fa)/1 -> Fout/1, Fin/1  "Fa(mol/min)"
  dT/dt/1 -> Kinetics/1(T_Reactor (K)), TemR/1, Scope/1, Sum6/2, Sum7/1  "Temp reactor (K)"
  Sum6/1 -> Hydrogen balance/1(T-Tref), Fout/3  "T-Tref"
  Tj/1 -> Sum7/2
  Jacket/1(Out1) -> Qjacket/1, Heat flow/3, energyJacket/1, Sum8/3  "Qjacket"
  Fin/1 -> Heat flow/2, energy Fi/1, Sum8/2  "Fin"
  Sum9/1 -> Heat flow/4, energy Fout/1, Sum8/4  "Fout"
  Energy dehydro/1(Qreact) -> Sum8/1, Heat flow/1, energy Rxn/1  "dREact"
  Sum8/1 -> Product8/1  "Tf-Tref"
  Product8/1 -> dT/dt/1  "dT/dt"
  Constant1/1 -> Fout/4
  TempFeed/1 -> dT/dt/2, Sum5/1
  Kinetics/1(Rateconstant) -> Product1/1  "(min-1)"
  Constant3/1 -> Fin/2
  CpH2 (kj/mol K @593K)/1 -> Hydrogen balance/3(CpH2)  "CpH2"
  Energy dehydro/2(F_molH2) -> Hydrogen balance/2(FmolH2)  "FmolH2 (mol/min)"
  Fout/1 -> Sum9/1  "Fout"
  Sum7/1 -> Jacket/1(In1)  "T-Tjacket"
  Hydrogen balance/1(QH2out) -> Sum9/2
  NACpA/1 -> Sum10/1  "dNh2"
  Sum10/1 -> Product8/2  "SumNiCpi"
  Hydrogen balance/2(N_h2*Cp) -> Sum10/2
  Mass balance A/1(Caout) -> Scope1/1, CA/1, Product1/2
  CA0 (mol/m3)/1 -> molar flow liquid (Fa)/2

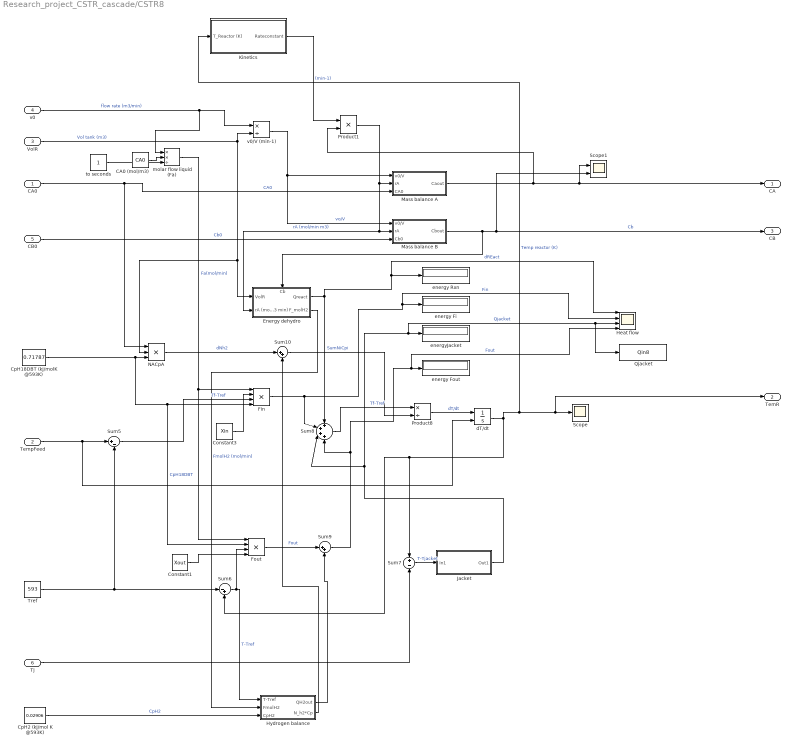
== system Research_project_CSTR_cascade/CSTR8 ==
  CA0 : Inport
  TempFeed : Inport  Port=2
  VolR : Inport  Port=3
  v0 : Inport  Port=4
  CB0 : Inport  Port=5
  Tj : Inport  Port=6
  CA0 (mol/m3) : Constant  Value=CA0
  Constant1 : Constant  Value=Xout
  Constant3 : Constant  Value=Xin
  CpH18DBT (kj/molK @593K) : Constant  Value=0.71787
  CpH2 (kj/mol K @593K) : Constant  Value=0.02906
  Energy dehydro : Subsystem
      settings: PortSchema="{\"entries\":[{\"content\":{\"sides\":[{\"content\":{\"connectorIds\":[\"In1\",\"In2\"]},\"type\":\"ConnectorPlacement.EquallySpacedRectSide\",\"uuid\":\"ea2ca829-97b9-403b-8ba1-0454ae3e30fe\"},{\"content\":{\"connectorIds\":[\"Out1\",\"Out2\"],\"side\":\"RIGHT\"},\"type\":\"ConnectorPlacement.EquallySpacedRectSide\",\"uuid\":\"58c9b242-3f0e-4d7f-8153-41ceacc042f7\"},{\"content\":{\"connectorIds\":[\"In3\"],\"side\":\"TOP\"},\"type\":\"ConnectorPlacement.EquallySpacedRectSide\",\"uuid\":\"130a98c9-d360-4861-8a60-9ab6de0c7020\"}]},\"type\":\"ConnectorPlacement.EquallySpacedConnector\",\"uuid\":\"a36fbf0c-f6b7-4cf9-83b8-7faebe270894\"}],\"packageUris\":[\"http://schema.mathworks.com/mf0/Connector/R2020b\"],\"version\":\"1.0\"}"
  Fin : Product  Inputs=4
  Fout : Product  Inputs=4
  Heat flow : Scope  NumInputPorts=4
  Hydrogen balance : Subsystem
  Jacket : Subsystem
  Kinetics : Subsystem
  Mass balance A : Subsystem
  Mass balance B : Subsystem
  NACpA : Product  Inputs=3
  Product1 : Product
  Product8 : Product  Inputs=*/
  Qjacket : ToWorkspace  VariableName=Qin8  SaveFormat=Timeseries  SampleTime=1
  Scope : Scope
  Scope1 : Scope  NumInputPorts=2
  Sum10 : Sum  Inputs=|++
  Sum5 : Sum  Inputs=|+-
  Sum6 : Sum  Inputs=|-+
  Sum7 : Sum  Inputs=+-
  Sum8 : Sum  Inputs=++++
  Sum9 : Sum  Inputs=|++
  Tref : Constant  Value=593
  dT/dt : Integrator  InitialConditionSource=external  InitialCondition=593
  energy Fi : Display
  energy Fout : Display
  energy Rxn : Display
  energyJacket : Display
  molar flow liquid (Fa) : Product  Inputs=**/
  to seconds : Constant
  v0/V (min-1) : Product  Inputs=*/
  CA : Outport
  TemR : Outport  Port=2
  CB : Outport  Port=3
  wires:
  VolR/1 -> Energy dehydro/1(VolR), NACpA/2, v0/V (min-1)/2  "Vol tank (m3)"
  v0/1 -> v0/V (min-1)/1, molar flow liquid (Fa)/1  "flow rate (m3/min)"
  CA0/1 -> NACpA/1, Mass balance A/3(CA0)  "CA0"
  Product1/1 -> Mass balance A/2(rA), Energy dehydro/2(rA (mol/m3 min)), Mass balance B/2(rA)  "rA (mol/min m3)"
  CB0/1 -> Mass balance B/3(Cb0)  "Cb0"
  v0/V (min-1)/1 -> Mass balance B/1(v0/V), Mass balance A/1(v0/V)  "vo/V"
  Mass balance B/1(Cbout) -> CB/1, Scope1/2, Energy dehydro/3(Cb)  "Cb"
  CpH18DBT (kj/molK @593K)/1 -> NACpA/3, Fin/4, Fout/2  "CpH18DBT"
  Tref/1 -> Sum5/2, Sum6/1
  Sum5/1 -> Fin/3  "Tf-Tref"
  to seconds/1 -> molar flow liquid (Fa)/3
  molar flow liquid (Fa)/1 -> Fout/1, Fin/1  "Fa(mol/min)"
  dT/dt/1 -> Kinetics/1(T_Reactor (K)), TemR/1, Scope/1, Sum6/2, Sum7/1  "Temp reactor (K)"
  Sum6/1 -> Hydrogen balance/1(T-Tref), Fout/3  "T-Tref"
  Tj/1 -> Sum7/2
  Jacket/1(Out1) -> Qjacket/1, Heat flow/3, energyJacket/1, Sum8/3  "Qjacket"
  Fin/1 -> Heat flow/2, energy Fi/1, Sum8/2  "Fin"
  Sum9/1 -> Heat flow/4, energy Fout/1, Sum8/4  "Fout"
  Energy dehydro/1(Qreact) -> Sum8/1, Heat flow/1, energy Rxn/1  "dREact"
  Sum8/1 -> Product8/1  "Tf-Tref"
  Product8/1 -> dT/dt/1  "dT/dt"
  Constant1/1 -> Fout/4
  TempFeed/1 -> dT/dt/2, Sum5/1
  Kinetics/1(Rateconstant) -> Product1/1  "(min-1)"
  Constant3/1 -> Fin/2
  CpH2 (kj/mol K @593K)/1 -> Hydrogen balance/3(CpH2)  "CpH2"
  Energy dehydro/2(F_molH2) -> Hydrogen balance/2(FmolH2)  "FmolH2 (mol/min)"
  Fout/1 -> Sum9/1  "Fout"
  Sum7/1 -> Jacket/1(In1)  "T-Tjacket"
  Hydrogen balance/1(QH2out) -> Sum9/2
  NACpA/1 -> Sum10/1  "dNh2"
  Sum10/1 -> Product8/2  "SumNiCpi"
  Hydrogen balance/2(N_h2*Cp) -> Sum10/2
  Mass balance A/1(Caout) -> Scope1/1, CA/1, Product1/2
  CA0 (mol/m3)/1 -> molar flow liquid (Fa)/2
